simulink model "Disturbance_Effect_on_OpenLoop_Vs_ClosedLoop"  (R2024a)
settings: Solver=VariableStepAuto  StartTime=0.0  StopTime=10.0  RelTol=1e-3
settings Model: Creator=VICTUS  LastModifiedBy=VICTUS

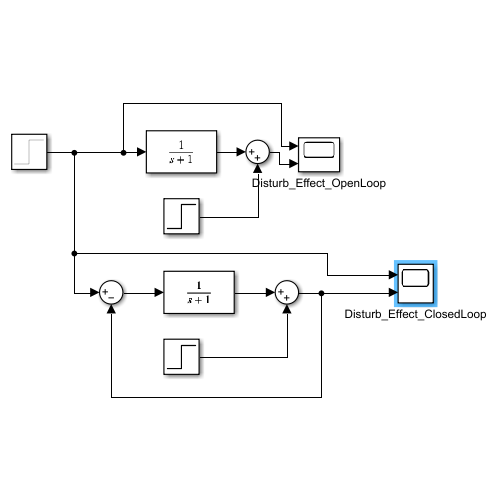
[thumbnail: Simulink's stored preview of the top-level diagram]
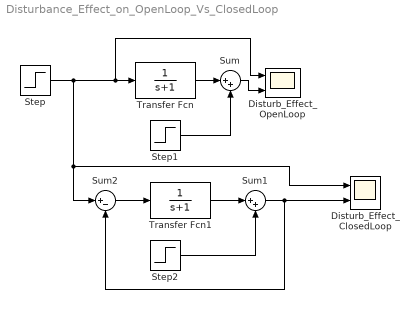
== system Disturbance_Effect_on_OpenLoop_Vs_ClosedLoop ==
  Disturb_Effect_ClosedLoop : Scope  NumInputPorts=2
  Disturb_Effect_OpenLoop : Scope  NumInputPorts=2
  Step : Step  SampleTime=0
  Step1 : Step  After=2  SampleTime=0
  Step2 : Step  After=2  SampleTime=0
  Sum : Sum  Inputs=|++
  Sum1 : Sum  Inputs=|++
  Sum2 : Sum  Inputs=|+-
  Transfer Fcn : TransferFcn  Denominator=[1 1]
  Transfer Fcn1 : TransferFcn  Denominator=[1 1]
  wires:
  Step/1 -> Disturb_Effect_OpenLoop/1, Transfer Fcn/1, Disturb_Effect_ClosedLoop/1, Sum2/1
  Transfer Fcn/1 -> Sum/1
  Step1/1 -> Sum/2
  Sum/1 -> Disturb_Effect_OpenLoop/2
  Transfer Fcn1/1 -> Sum1/1
  Step2/1 -> Sum1/2
  Sum2/1 -> Transfer Fcn1/1
  Sum1/1 -> Sum2/2, Disturb_Effect_ClosedLoop/2
